simulink model "RL_Project"  (R2023b)
settings: Solver=FixedStepAuto  StartTime=0.0  StopTime=75  FixedStep=0.025  RelTol=1e-3
model workspace (MAT data in the model file):
  A : Simulink.Parameter (value not decoded)
  Aag : Simulink.Parameter (value not decoded)
  B : Simulink.Parameter (value not decoded)
  Bag : Simulink.Parameter (value not decoded)
  C : Simulink.Parameter (value not decoded)
  Cag : Simulink.Parameter (value not decoded)
  uang = [0 0 0 0 0 0 5.50670620214e-14 5.44009282066e-14 0 -3.99756362155e-05 -2.83106871279e-14 0 ... (9003 elements, 3x3001)]
  upos = [0 0 0 5.62466739851e-14 5.62327961973e-14 0 -2.39975660277e-05 4.94743135349e-14 0 -9.31686537426e-05 7.62168106405e-14 0 ... (9003 elements, 3x3001)]
values from neighbouring files (symbols this model uses):
  alpha = 0.5    [RL_iteration.m]    (also in RL_iteration2.m; train_AQLRL.m = max(alpha * alpha_decay, alpha_min))
  gamma = 0.9    [RL_iteration.m]    (also in RL_iteration2.m; train_AQLRL.m = 0.5)
  ref = [0 0 1.5 -3.29206127203e-06 0.00314263790126 1.5 -1.31682306379e-05 0.00628526200819 1.5 -2.96284647472e-05 0.00942785852649 1.5 ... (9000 elements, 3x3000)]    [circulartrajectory.mat]    (also in generate_circ_trajectory.m = [x;y;z]; generate_sprial_trajectory.m = [x;y;z]; generate_triangle_trajectory.m = [x;y;z]; spiralTrajectory.mat = [0 0 1.5 -2.96284647472e-05 0.00942785852649 1.50050016672 -)
undefined symbols (not defined in the file or in its folder): Qang_lastiter, Qpos_lastiter
libraries: aerolibanimutils x1
(part 2 of 2)

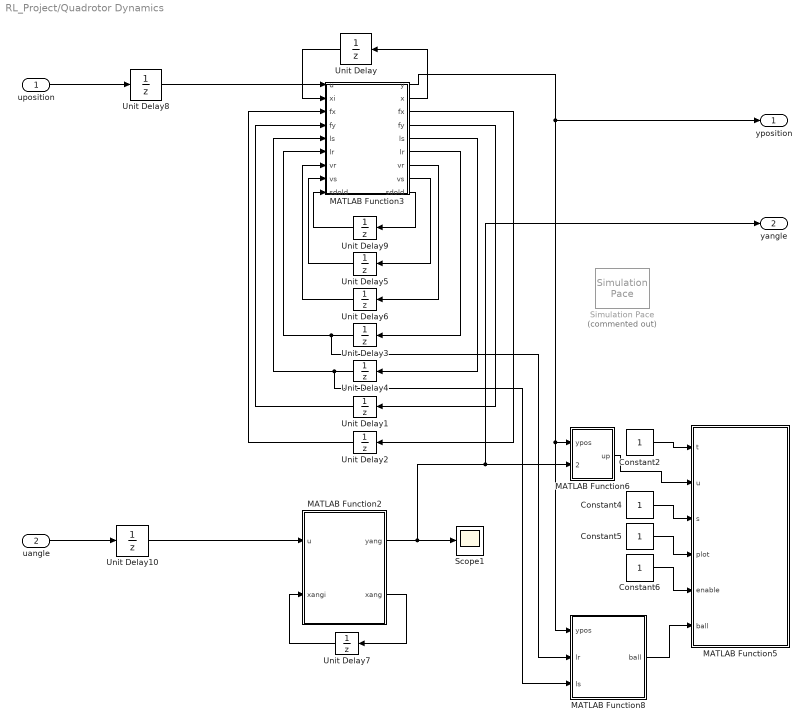
== system RL_Project/Quadrotor Dynamics ==
  uposition : Inport
  uangle : Inport  Port=2
  Constant{2,4..6} (4 alike) : Constant
  MATLAB Function2 : MATLAB Function  TreatAsAtomicUnit=on
  MATLAB Function3 : MATLAB Function  TreatAsAtomicUnit=on
  MATLAB Function5 : MATLAB Function  TreatAsAtomicUnit=on
  MATLAB Function6 : MATLAB Function  TreatAsAtomicUnit=on
  MATLAB Function8 : MATLAB Function  TreatAsAtomicUnit=on
  Scope1 : Scope
  Simulation Pace : aerolibanimutils/Simulation Pace  Commented=on  SimulationPace=1  SleepMode=Auto  OutputPaceError=off  SampleTime=-1
  Unit Delay : UnitDelay  InitialCondition=|  SampleTime=-1  HasFrameUpgradeWarning=on
      | [0
      | 0
      | 0
      | 0
      | 1.50000000000000
      | 0]
  Unit Delay{1..6,9} (7 alike) : UnitDelay  SampleTime=-1  HasFrameUpgradeWarning=on
  Unit Delay10 : UnitDelay  InitialCondition=|  SampleTime=-1  HasFrameUpgradeWarning=on
      | [0
      | 0
      | 0]
  Unit Delay7 : UnitDelay  InitialCondition=|  SampleTime=-1  HasFrameUpgradeWarning=on
      | [0
      | 0
      | 0
      | 0
      | 0
      | 0]
  Unit Delay8 : UnitDelay  InitialCondition=|  SampleTime=-1  HasFrameUpgradeWarning=on
      | [0
      | 0
      | 0]
  yposition : Outport
  yangle : Outport  Port=2
  wires:
  Unit Delay6/1 -> MATLAB Function3/7("vr ")
  MATLAB Function3/2(x) -> Unit Delay/1
  MATLAB Function3/5(ls) -> Unit Delay4/1
  MATLAB Function2/1(yang) -> Scope1/1, yangle/1, MATLAB Function6/2(yang)
  Constant4/1 -> MATLAB Function5/3(s)
  Constant2/1 -> MATLAB Function5/1(t)
  MATLAB Function3/4(fy) -> Unit Delay1/1
  Unit Delay/1 -> MATLAB Function3/2(xi)
  MATLAB Function3/9(sdold) -> Unit Delay9/1
  MATLAB Function8/1(ball) -> MATLAB Function5/6(ball)
  Unit Delay4/1 -> MATLAB Function8/3(ls), MATLAB Function3/5("ls ")
  Unit Delay2/1 -> MATLAB Function3/3("fx ")
  MATLAB Function2/2(xang) -> Unit Delay7/1
  MATLAB Function3/1(y) -> yposition/1, MATLAB Function8/1(ypos), MATLAB Function6/1(ypos)
  MATLAB Function3/6(lr) -> Unit Delay3/1
  Constant5/1 -> MATLAB Function5/4(plot)
  MATLAB Function3/8(vs) -> Unit Delay5/1
  Unit Delay3/1 -> MATLAB Function8/2(lr), MATLAB Function3/6("lr ")
  Unit Delay5/1 -> MATLAB Function3/8("vs ")
  Constant6/1 -> MATLAB Function5/5(enable)
  MATLAB Function6/1(up) -> MATLAB Function5/2(u)
  Unit Delay7/1 -> MATLAB Function2/2(xangi)
  MATLAB Function3/7(vr) -> Unit Delay6/1
  MATLAB Function3/3(fx) -> Unit Delay2/1
  Unit Delay9/1 -> MATLAB Function3/9("sdold ")
  Unit Delay1/1 -> MATLAB Function3/4("fy ")
  uposition/1 -> Unit Delay8/1
  uangle/1 -> Unit Delay10/1
  Unit Delay8/1 -> MATLAB Function3/1(u)
  Unit Delay10/1 -> MATLAB Function2/1(u)

== matlab function RL_Project/Quadrotor Dynamics/MATLAB Function6 ==
  data: up output; ypos input; yang input
function up= upp(ypos,yang)
up = [ypos(1) -ypos(2) -ypos(3) yang(1) yang(2) yang(3)];

== matlab function RL_Project/Quadrotor Dynamics/MATLAB Function8 ==
  data: ball output; ypos input; lr input; ls input
function ball= balll(ypos,lr,ls)
ball=[ypos(1)+lr(1) -(ypos(2)+ls(1)) 1-ypos(3)-sqrt(0.25-lr(1)^2-ls(1)^2)]';

== matlab function RL_Project/MATLAB Function1 ==
  data: State input; action output; Reward input; alpha parameter; gamma parameter; Qpos_lastiter parameter; Q_pos output; Q_ang output; Qang_lastiter parameter; Qpos_tminus input; Qang_tminus input
function [action,Q_pos, Q_ang] = fcn(State, Reward, alpha, gamma, Qpos_lastiter, Qang_lastiter, Qpos_tminus, Qang_tminus)
    
    action = zeros(1,6); 
    Q_pos = zeros(50, 50, 3, 5, 5, 5); 
    Q_ang = zeros(50, 50, 3, 3, 3, 3);


    % discretize current state
    s = getStateIndex(State); 
    % choose action using epsilon greedy method
    epsilon = 0.1; 
    if rand < epsilon
        pos_action = sampleRandomPosAction(); % Exploration
    else 
        pos_action = selectBestPosAction(Qpos_lastiter, s); %Exploitation
    end 

    if rand < epsilon
        ang_action = sampleRandomAngAction(); 
    else
        ang_action = selectBestAngAction(Qang_lastiter, s); 
    end 
    
    action = [pos_action, ang_action]; 


    % convert chosen action to index
    apos = getPosActionIndex(pos_action); 
    aang = getAngActionIndex(ang_action); 

    % get current Q value and max Q value for next state
    Qpos_current = Qpos_lastiter(s(1), s(2), s(3), apos(1), apos(2), apos(3)); 
    Qang_current = Qang_lastiter(s(1), s(2), s(3), aang(1), aang(2), aang(3)); 


    Qpos_max_next = maxPosQNextState(Qpos_tminus, s); 
    Qang_max_next = maxAngQNextState(Qang_tminus, s); 



    % Q-learning update
    Qpos_updated = Qpos_current + alpha * (Reward + gamma * Qpos_max_next - Qpos_current); 
    Qang_updated = Qang_current + alpha * (Reward + gamma * Qang_max_next - Qang_current); 

    % Update the Q Matrix
    Q_pos = Qpos_lastiter; 
    Q_ang = Qang_lastiter; 
    Q_pos(s(1), s(2), s(3), apos(1), apos(2), apos(3)) = Qpos_updated; 
    Q_ang(s(1), s(2), s(3), aang(1), aang(2), aang(3)) = Qang_updated; 
    

   
function idx = getStateIndex(state)
    % New discretization settings
    pos_bins_x = 50; 
    pos_bins_y = 50; 
    pos_bins_z = 3; 

    state_min = [-1, -1, 0]; 
    state_max = [2, 2, 2]; 

    idx = zeros(1,3); 
    idx(1) = floor((state(1) - state_min(1)) / (state_max(1) - state_min(1)) * (pos_bins_x-1)) + 1; 
    idx(2) = floor((state(2) - state_min(2)) / (state_max(2) - state_min(2)) * (pos_bins_y-1)) + 1; 
    idx(3) = floor((state(3) - state_min(3)) / (state_max(3) - state_min(3)) * (pos_bins_z-1)) + 1; 

    idx = max(min(idx, [pos_bins_x, pos_bins_y, pos_bins_z]),1); 

end

    function idx = getPosActionIndex(action)
        bins_pos = [-0.02, -0.01, 0, 0.01, 0.02]; 
        idx = zeros(1,3); 
        for i = 1:3
            [~, idx(i)] = min(abs(action(i)-bins_pos)); 
        end 
    end 

    function idx = getAngActionIndex(action)
        bins_ang = [-0.01, 0, 0.01]; 
        idx = zeros(1,3); 
        for i = 1:3 
            [~, idx(i)] = min(abs(action(i) - bins_ang)); 
        end 
    end 


function pos_action = sampleRandomPosAction()
        bins_pos = [-0.02, -0.01, 0, 0.01, 0.02]; 
        pos_action = bins_pos(randi(length(bins_pos), 1,3)); 
        
end 

function ang_action = sampleRandomAngAction()
    bins_ang = [-0.01, 0, 0.01]; 
    ang_action = bins_ang(randi(length(bins_ang), 1, 3)); 

end 


    function best_pos_action = selectBestPosAction(Q, s)
        bins_pos = [-0.02, -0.01, 0, 0.01, 0.02]; 
        maxQ = -Inf; 
        best_idx = [1,1,1]; 
        for a1 = 1:5
            for a2 = 1:5
                for a3 = 1:5
                    q = Q(s(1), s(2), s(3), a1, a2, a3); 
                    if q > maxQ
                        maxQ = q; 
                        best_idx = [a1, a2, a3]; 
                    end 
                end
            end
        end
        best_pos_action = [bins_pos(best_idx(1)), bins_pos(best_idx(2)), bins_pos(best_idx(3))]; 
    
    end 

    function best_ang_action = selectBestAngAction(Q,s)
        bins_ang = [-0.01, 0, 0.01]; 
        maxQ = -Inf; 
        best_idx = [1,1,1]; 
        for a1 = 1:3
            for a2 = 1:3
                for a3 = 1:3
                    q = Q(s(1), s(2), s(3), a1, a2,a3); 
                    if q > maxQ
                        maxQ = q; 
                        best_idx = [a1, a2, a3]; 
                    end 
                end 
            end
        end
        best_ang_action = [bins_ang(best_idx(1)), bins_ang(best_idx(2)), bins_ang(best_idx(3))]; 
    
    end 



    function maxQ = maxPosQNextState(Q,s)
        maxQ = -Inf; 
        for a1 = 1:5
            for a2 = 1:5
                for a3 = 1:5
                    q = Q(s(1), s(2), s(3), a1, a2, a3); 
                    if q > maxQ
                        maxQ = q; 
                    end 
                end
            end
        end 
    end 

    function maxQ = maxAngQNextState(Q,s)
        maxQ = -Inf; 
        for a1 = 1:3
            for a2 = 1:3
                for a3 = 1:3
                    q = Q(s(1), s(2), s(3), a1, a2, a3); 
                    if q > maxQ
                        maxQ = q; 
                    end 
                end 
            end 
        end 
    end 

 
end

== matlab function RL_Project/MATLAB Function ==
  data: state input; action input; reward output; y input
function reward  = fcn(state, action, y)
    action = action(:).'; 
    % Define weights
    pos_weight = [100, 100, 20];
    ang_weight = [10, 10, 10];
    action_weight = [0.1, 0.1, 0.1, 0.05, 0.05, 0.05];

    % Split state and ref
    pos_state = state(1:3);
    ang_state = state(4:6);
    pos_ref = y(1:3);
    ang_ref = y(4:6);

    % Errors
    pos_error = (pos_state - pos_ref).^2;
    ang_error = (ang_state - ang_ref).^2;
    action_penalty = (action).^2;

    % Proper summing
    reward = - sum( sum(pos_weight .* pos_error) ...
               + sum(ang_weight .* ang_error) ...
               + sum(action_weight .* action_penalty) );

== matlab function RL_Project/MATLAB Function3 ==
  data: ref input; y output; t input
function y = fcn(ref, t)
T = floor(t/0.025)+1;
y = ref(:,T);

== matlab function RL_Project/Quadrotor Dynamics/MATLAB Function2 ==
  data: yang output; xang output; u input; xangi input
function [yang,xang]= sysang(u,xangi)
Ts = 1/40;
g = 9.81;
A = [1,0.0250000000000000,0,0,0,0;0,1,0,0,0,0;0,0,1,0.0250000000000000,0,0;0,0,0,1,0,0;0,0,0,0,1,0.0250000000000000;0,0,0,0,0,1];
B = [0.0416666666666667,0,0;3.33333333333333,0,0;0,0.0416666666666667,0;0,3.33333333333333,0;0,0,0.0240384615384615;0,0,1.92307692307692];
C = [1,0,0,0,0,0;0,0,1,0,0,0;0,0,0,0,1,0];
D = zeros(3,3);
xang = zeros(6,1);
yang = zeros(3,1);
xang = A*xangi + B*u;
yang = C*xang + D*u;

== matlab function RL_Project/Quadrotor Dynamics/MATLAB Function3 ==
  data: y output; x output; u input; xi input; fx input; fy input; fx output; fy output; ls input; lr input; ls output; lr output; vr input; vs input; vr output; vs output; sdold input; sdold output
function [y,x, fx,fy,ls,lr,vr,vs,sdold]= syspos(u,xi,fx,fy,ls,lr,vr,vs,sdold)
Ts = 1/40;
g = 9.81;
A = [1 0.025 0 0 0 0;0 1 0 0 0 0;0 0 1 0.025 0 0;0 0 0 1 0 0;0 0 0 0 1 0.025;0 0 0 0 0 1];
B = [-0.003065625 0 0;-0.24525 0 0;0 0.003065625 0;0 0.24525 0;0 0 0.0003125;0 0 0.025];
C = [1 0 0 0 0 0;0 0 1 0 0 0;0 0 0 0 1 0];
D = zeros(3,3);
x = zeros(6,1);
y = zeros(3,1);
x = A*xi + B*u;
y = C*x + D*u;
x(2) = x(2) - fx;
x(4) = x(4) - fy;


xdold = x(2)-xi(2);
ydold = x(4)-xi(4);
zdold = x(6)-xi(6);

yita = sqrt(0.5^2-lr^2-ls^2);
vrold = vr;
vsold = vs;
vr = ( yita^4*xdold - lr*yita^3*zdold + lr*ls*yita^2*sdold +...
    (lr*0.5^2-lr*ls^2)*vr^2 +...
    (lr*0.5^2-lr^3)*vs^2 +...
    2*vr*vs*lr^2*ls + lr*g*yita^3 )/((ls^2-0.5^2)*yita^2);
lr = lr + vr*Ts;
rdold = vr-vrold;

vs = ( yita^4*ydold - ls*yita^3*zdold + lr*ls*yita^2*rdold +...
    (ls*0.5^2-ls*lr^2)*vs^2 +...
    (ls*0.5^2-ls^3)*vr^2 +...
    2*vr*vs*ls^2*lr + ls*g*yita^3 )/((lr^2-0.5^2)*yita^2);
ls = ls + vs*Ts;
% sdold = vs(1,i+1);
sdold = vs(1)-vsold(1);

fx = 0.3*(xdold+rdold);
fy = 0.3*(ydold+sdold);

== matlab function RL_Project/Quadrotor Dynamics/MATLAB Function5 ==
  data: t input; u input; s input; plot input; enable input; ball input
function qd_plot(t,u,s, plot, enable,ball)
    quad.nrotors =4;
    quad.d = 0.17;
    quad.r = 0.1;
    
    a1s = zeros(1, quad.nrotors);
    b1s = zeros(1, quad.nrotors);

    
    % vehicle dimensons
    d = quad.d; %Hub displacement from COG
    r = quad.r; %Rotor radius
    D = zeros(3,4);
    C = zeros(3,4);
    for i = 1:quad.nrotors
        theta = (i-1)/quad.nrotors*2*pi;
        %   Di      Rotor hub displacements (1x3)
        % first rotor is on the x-axis, clockwise order looking down from above
        D(:,i) = [ d*cos(theta); d*sin(theta); 0];
%         scal = s(1)/4;
        scal = 0.2/4;
        %Attitude center displacements
        C(:,i) = [ scal*cos(theta); scal*sin(theta); 0];
    end
    
    if enable == 1
        %draw ground
        figure(1);
        clf;
        if length(s) == 1
            axis([-0.5 1.5 -0.5 1.5 0 2]);
        else
%             axis([-s(1) s(1) -s(1) s(1) 0 s(2)])
            axis([-0.5 s(1) -0.5 s(1) 0 s(2)])
            s = 1.5;
        end
        hold on;
        
        % plot the ground boundaries and the big cross
        plot3([-0.5 -0.5],[-0.5 1],[0 0],'-b')
        plot3([-0.5 1.5],[-0.5 -0.5],[0 0],'-b')
        plot3([-0.5 1.5],[-0.5 1.5],[0 0],'-b')
        plot3([1.5 -0.5],[1.5 1.5],[0 0],'-b')
        plot3([1.5 1.5],[1.5 -0.5],[0 0],'-b')
        plot3([-0.5 1.5],[1.5 -0.5],[0 0],'-b')
        
        plot3([0 1], [0 0], [1.5 1.5],':r','LineWidth',0.2)
        plot3([1 1], [0 1], [1.5 1.5],':r','LineWidth',0.2)
        plot3([0 1], [1 1], [1.5 1.5],':r','LineWidth',0.2)
        plot3([0 0], [0 1], [1.5 1.5],':r','LineWidth',0.2)
        
        plot3([0 1], [0 0], [1 1],':r','LineWidth',0.2)
        plot3([1 1], [0 1], [1 1],':r','LineWidth',0.2)
        plot3([0 1], [1 1], [1 1],':r','LineWidth',0.2)
        plot3([0 0], [0 1], [1 1],':r','LineWidth',0.2)
        %READ STATE
        z = [u(1);u(2);u(3)];
        n = [u(4);u(5);u(6)];
        
        %PREPROCESS ROTATION MATRIX
        phi = n(1);    %Euler angles
        the = n(2);
        psi = n(3);
        
        R = [cos(the)*cos(phi) sin(psi)*sin(the)*cos(phi)-cos(psi)*sin(phi) cos(psi)*sin(the)*cos(phi)+sin(psi)*sin(phi);   %BBF > Inertial rotation matrix
            cos(the)*sin(phi) sin(psi)*sin(the)*sin(phi)+cos(psi)*cos(phi) cos(psi)*sin(the)*sin(phi)-sin(psi)*cos(phi);
            -sin(the)         sin(psi)*cos(the)                            cos(psi)*cos(the)];
        
        %Manual Construction
        %Q3 = [cos(psi) -sin(psi) 0;sin(psi) cos(psi) 0;0 0 1];   %Rotation mappings
        %Q2 = [cos(the) 0 sin(the);0 1 0;-sin(the) 0 cos(the)];
        %Q1 = [1 0 0;0 cos(phi) -sin(phi);0 sin(phi) cos(phi)];
        %R = Q3*Q2*Q1;    %Rotation matrix
        
        %CALCULATE FLYER TIP POSITONS USING COORDINATE FRAME ROTATION
        F = [1 0 0;0 -1 0;0 0 -1];
        
        %Draw flyer rotors
        t = [0:pi/8:2*pi];
        circle = zeros(3,17);
        for j = 1:length(t)
            circle(:,j) = [r*sin(t(j));r*cos(t(j));0];
        end
        hub = zeros(3,4);
        tippath = zeros(3,17,4);
        for i = 1:quad.nrotors
            hub(:,i) = F*(z + R*D(:,i)); %points in the inertial frame
            center = F*z;
            ball_pos = F*ball;
            plot3(center(1),center(2),center(3),'r.')
            plot3(ball_pos(1),ball_pos(2),ball_pos(3),'co')
            plot3([center(1) ball_pos(1)],[center(2) ball_pos(2)],[center(3) ball_pos(3)],'-b')
            
            q = 1; %Flapping angle scaling for output display - makes it easier to see what flapping is occurring
            Rr = [cos(q*a1s(i))  sin(q*b1s(i))*sin(q*a1s(i)) cos(q*b1s(i))*sin(q*a1s(i));   %Rotor > Plot frame
                0              cos(q*b1s(i))               -sin(q*b1s(i));
                -sin(q*a1s(i)) sin(q*b1s(i))*cos(q*a1s(i)) cos(q*b1s(i))*cos(q*a1s(i))];
            
            tippath(:,:,i) = F*R*Rr*circle;
            plot3([hub(1,i)+tippath(1,:,i)],[hub(2,i)+tippath(2,:,i)],[hub(3,i)+tippath(3,:,i)],'b-')
        end
        
        %Draw flyer
        hub0 = F*z;  % centre of vehicle
        for i = 1:quad.nrotors
            % line from hub to centre plot3([hub(1,N) hub(1,S)],[hub(2,N) hub(2,S)],[hub(3,N) hub(3,S)],'-b')
            plot3([hub(1,i) hub0(1)],[hub(2,i) hub0(2)],[hub(3,i) hub0(3)],'-b')
            
            % plot a circle at the hub itself
            plot3([hub(1,i)],[hub(2,i)],[hub(3,i)],'o')
        end
        
        % plot the vehicle's centroid on the ground plane
        plot3([z(1) 0],[-z(2) 0],[0 0],'--k')
        plot3([z(1)],[-z(2)],[0],'xk')
        plot3([z(1) z(1)],[-z(2) -s],[0 0],'r-.')

        % label the axes
        xlabel('x');
        ylabel('y');
        zlabel('z (height above ground)');
        view([-5 -2 5]);
    end;
